simulink model "verification_simulink"  (R2015a)
settings: Solver=ode3  StartTime=0.0  StopTime=T_sim_length  FixedStep=T_sim  RelTol=1e-3
values from neighbouring files (symbols this model uses):
  Ad = sys_discrete.a + L * C + sys_discrete.b * K    [example_integrator.m]    (also in param_pendulum_calc.m)
  Ap = [0, 1; 0, 0]    [example_integrator.m]    (also in param_pendulum.m = [0, 1; upright * omega0 ^ 2, -2 * xi * omega0])
  Bd = -L    [example_integrator.m]    (also in param_pendulum_calc.m)
  Bp = [0; 1]    [example_integrator.m]    (also in example_mimo.m = [Bp, Bp]; param_pendulum.m = [0; omega0 / 9.81])
  C = [1, 0]    [example_integrator.m]    (also in example_mimo.m = [C; C]; param_pendulum.m)
  Cd = K    [example_integrator.m]    (also in param_pendulum_calc.m)
  delay_u_sim_is_random = 0    [example_integrator.m]    (also in example_pendulum_static_delay.m = false; example_pendulum_varying_delay.m = false; param_pendulum_timevarying.m = false)
  delay_y_sim_is_random = 0    [example_integrator.m]    (also in example_pendulum_static_delay.m = false; example_pendulum_varying_delay.m = true; param_pendulum_timevarying.m = false)
  Gp = [0; 1]    [example_integrator.m]    (also in param_pendulum.m)
  N_p = 1e-2    (= 0.01)    [example_integrator.m]    (also in example_mimo.m = blkdiag(N_p, N_p) * 2; param_pendulum.m = 1e-06)
  Q_tilde = [0.00968, 0; 0, 0.0470]    [example_integrator.m]    (also in param_pendulum.m = 550 * eye(2))
  R_tilde = 0.768    [example_integrator.m]    (also in example_mimo.m = blkdiag(R_tilde, R_tilde) * 2; param_pendulum.m = 0.8)
  T = 1    [example_integrator.m]    (also in param_pendulum.m = 0.2)
  T_sim = T * 1e-3    (= 0.001)    [example_integrator.m]    (also in param_pendulum.m = 0.0001)
libraries: simulink x9, dspsigops x2
settings Model: ExtModeTrigDuration=100  Creator=ak22emur  LastModifiedBy=ak22emur
settings DataIOCC: LimitDataPoints=off  SaveFormat=StructureWithTime  SaveOutput=off  SignalLogging=off  DSMLogging=off  VisualizeSimOutput=off  SaveTime=off  StateSaveName=tmp_raccel_xout  SignalLoggingName=tmp_raccel_logsout
settings OptimizationCC: InlineParams=on  InlineInvariantSignals=on  EfficientMapNaN2IntZero=off  SimCompilerOptimization=on
settings HardwareCC: TargetLongLongMode=on  TargetIntDivRoundTo=Zero  TargetEndianess=LittleEndian  TargetHWDeviceType=MATLAB Host  ProdEqTarget=off
settings RTWCC: SystemTargetFile=raccel.tlc  TemplateMakefile=raccel_default_tmf  RTWVerbose=off  RTWUseSimCustomCode=on
settings CodeAppCC: GenerateComments=off  MaxIdLength=128  SimulinkBlockComments=off
settings RaccelTargetCC: ERTMultiwordTypeDef=System defined  ERTMultiwordLength=256  GeneratePreprocessorConditionals=Disable all  ERTFirstTimeCompliant=off  MultiInstanceERTCode=off  ENABLE_SLEXEC_SSBRIDGE=0  RTWCAPIParams=off

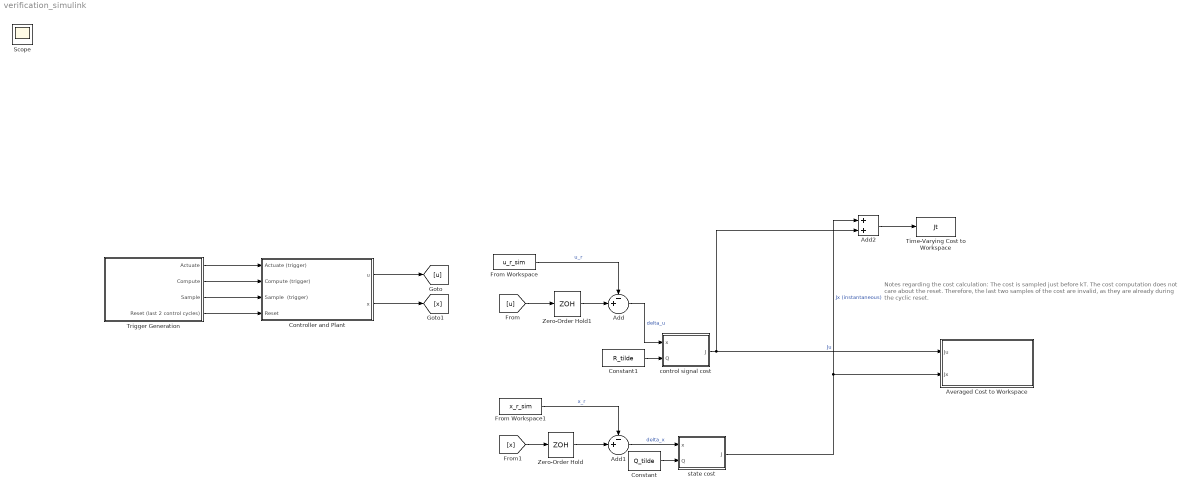
== system verification_simulink ==
  note: Notes regarding the cost calculation:
      | The cost is sampled just before kT.
      | The cost computation does not care about the reset. Therefore, the last two samples of the cost are invalid, as they are already during the cyclic reset.
  Add : Sum  Inputs=-+|
  Add1 : Sum  Inputs=-+|
  Add2 : Sum
  Averaged Cost to Workspace : Subsystem
  Constant : Constant  Value=Q_tilde
  Constant1 : Constant  Value=R_tilde
  Controller and Plant : Subsystem
  From Workspace : FromWorkspace  VariableName=u_r_sim  SampleTime=T  Interpolate=off  OutputAfterFinalValue=Cyclic repetition
  From Workspace1 : FromWorkspace  VariableName=x_r_sim  SampleTime=T  Interpolate=off  OutputAfterFinalValue=Cyclic repetition
  Time-Varying Cost to Workspace : ToWorkspace  VariableName=Jt  SampleTime=T
  Trigger Generation : Subsystem
  Zero-Order Hold : ZeroOrderHold  SampleTime=T
  Zero-Order Hold1 : ZeroOrderHold  SampleTime=T
  control signal cost : MATLAB Function  TreatAsAtomicUnit=on
  state cost : MATLAB Function  TreatAsAtomicUnit=on
  Scope : Scope
      settings: YMin=0  YMax=1.4
  wires:
  Constant/1 -> state cost/2(Q)
  state cost/1(J) -> Averaged Cost to Workspace/2(Jx), Add2/1  "Jx (instantaneous)"
  Constant1/1 -> control signal cost/2(Q)
  control signal cost/1(J) -> Add2/2, Averaged Cost to Workspace/1(Ju)  "Ju"
  [u] -> Zero-Order Hold1/1
  Add2/1 -> Time-Varying Cost to Workspace/1
  Trigger Generation/1(Actuate) -> Controller and Plant/1(Actuate (trigger))
  Trigger Generation/2(Compute) -> Controller and Plant/2(Compute (trigger))
  Trigger Generation/3(Sample) -> Controller and Plant/3(Sample  (trigger))
  Controller and Plant/1(u) -> [u]
  Controller and Plant/2(x) -> [x]
  Trigger Generation/4(Reset (last 2 control cycles)) -> Controller and Plant/4(Reset)
  Add/1 -> control signal cost/1(x)  "delta_u"
  Zero-Order Hold1/1 -> Add/2
  From Workspace/1 -> Add/1  "u_r"
  Add1/1 -> state cost/1(x)  "delta_x"
  [x] -> Zero-Order Hold/1
  From Workspace1/1 -> Add1/1  "x_r"
  Zero-Order Hold/1 -> Add1/2

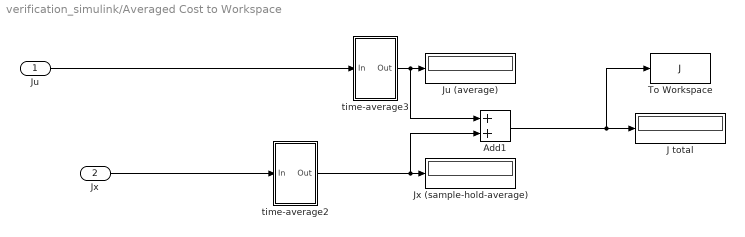
== system verification_simulink/Averaged Cost to Workspace ==
  Ju : Inport
  Jx : Inport  Port=2
  Add1 : Sum
  J total : Display
  Ju (average) : Display
  Jx (sample-hold-average) : Display
  To Workspace : ToWorkspace  VariableName=J  SampleTime=-1
      settings: MaxDataPoints=1
  time-average2 : Subsystem
  time-average3 : Subsystem
  wires:
  time-average3/1(Out) -> Add1/1, Ju (average)/1
  Add1/1 -> To Workspace/1, J total/1
  time-average2/1(Out) -> Add1/2, Jx (sample-hold-average)/1
  Ju/1 -> time-average3/1(In)
  Jx/1 -> time-average2/1(In)

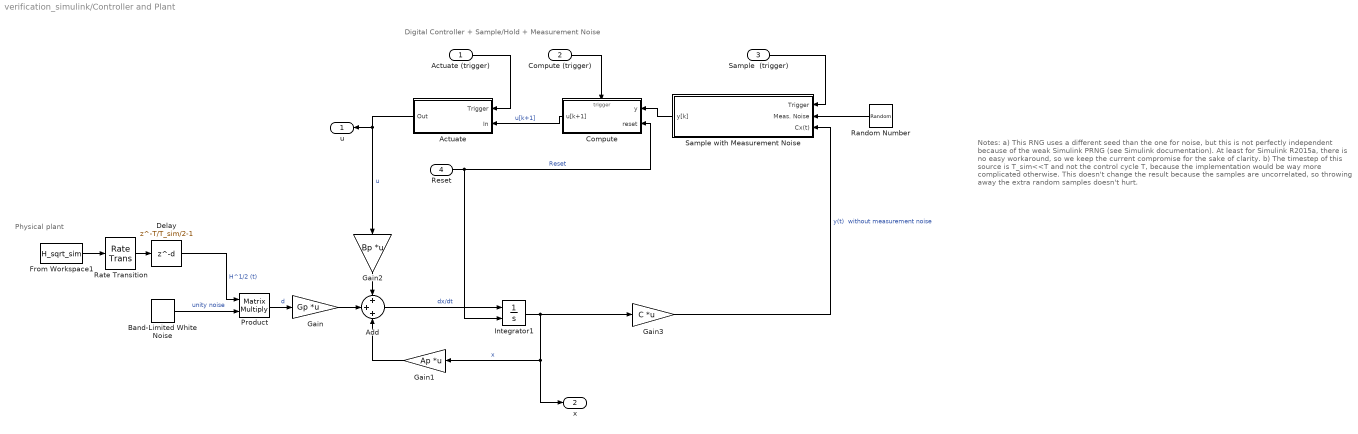
== system verification_simulink/Controller and Plant ==
  note: Digital Controller + Sample/Hold + Measurement Noise
  note: Physical plant
  note: Notes:
      | a) This RNG uses a different seed than the one for noise,
      | but this is not perfectly independent because of the weak Simulink PRNG
      | (see Simulink documentation).
      | At least for Simulink R2015a, there is no easy workaround, so we keep the current compromise for the sake of clarity.
      | b) The timestep of this source is T_sim<<T and not the control cycle T, because the implementation would be way more complicated otherwise.
      | This doesn't change the result because the samples are uncorrelated, so throwing away the extra random samples doesn't hurt.
  Actuate (trigger) : Inport
  Compute (trigger) : Inport  Port=2
  Sample  (trigger) : Inport  Port=3
  Reset : Inport  Port=4
  Actuate : Subsystem  TreatAsAtomicUnit=on
  Add : Sum  Inputs=+++
  Band-Limited White Noise : simulink/Sources/Band-Limited White Noise  Cov=ones(size(Gp,2), 1)  Ts=T_sim  seed=[23341]
  Compute : Subsystem  TreatAsAtomicUnit=on
  Delay : Delay  DelayLength=T/T_sim/2-1
  From Workspace1 : FromWorkspace  VariableName=H_sqrt_sim  SampleTime=T  Interpolate=off  OutputAfterFinalValue=Cyclic repetition
  Gain : Gain  Gain=Gp  Multiplication=Matrix(K*u)
  Gain1 : Gain  Gain=Ap  Multiplication=Matrix(K*u)
  Gain2 : Gain  Gain=Bp  Multiplication=Matrix(K*u)
  Gain3 : Gain  Gain=C  Multiplication=Matrix(K*u)
  Integrator1 : Integrator  ExternalReset=level
  Product : Product  Multiplication=Matrix(*)
  Random Number : RandomNumber  Variance=diag(N_p)  Seed=13379812+[1:length(N_p)]  SampleTime=T_sim
  Rate Transition : RateTransition
  Sample with Measurement Noise : Subsystem  TreatAsAtomicUnit=on
  u : Outport
  x : Outport  Port=2
  wires:
  Gain3/1 -> Sample with Measurement Noise/3(Cx(t))  "y(t)  without measurement noise"
  Gain/1 -> Add/2
  Add/1 -> Integrator1/1  "dx/dt"
  Actuate/1(Out) -> u/1, Gain2/1  "u"
  Gain2/1 -> Add/1
  Compute (trigger)/1 -> Compute/Trigger
  Actuate (trigger)/1 -> Actuate/1(Trigger)
  Integrator1/1 -> x/1, Gain1/1, Gain3/1  "x"
  Compute/1(u[k+1]) -> Actuate/2(In)  "u[k+1]"
  Gain1/1 -> Add/3
  Reset/1 -> Compute/2(reset), Integrator1/2  "Reset"
  Sample  (trigger)/1 -> Sample with Measurement Noise/1(Trigger)
  Random Number/1 -> Sample with Measurement Noise/2(Meas. Noise)
  Sample with Measurement Noise/1(y[k]) -> Compute/1(y)
  Product/1 -> Gain/1  "d"
  Band-Limited White Noise/1 -> Product/2  "unity noise"
  From Workspace1/1 -> Rate Transition/1
  Rate Transition/1 -> Delay/1
  Delay/1 -> Product/1  "H^1/2 (t)"

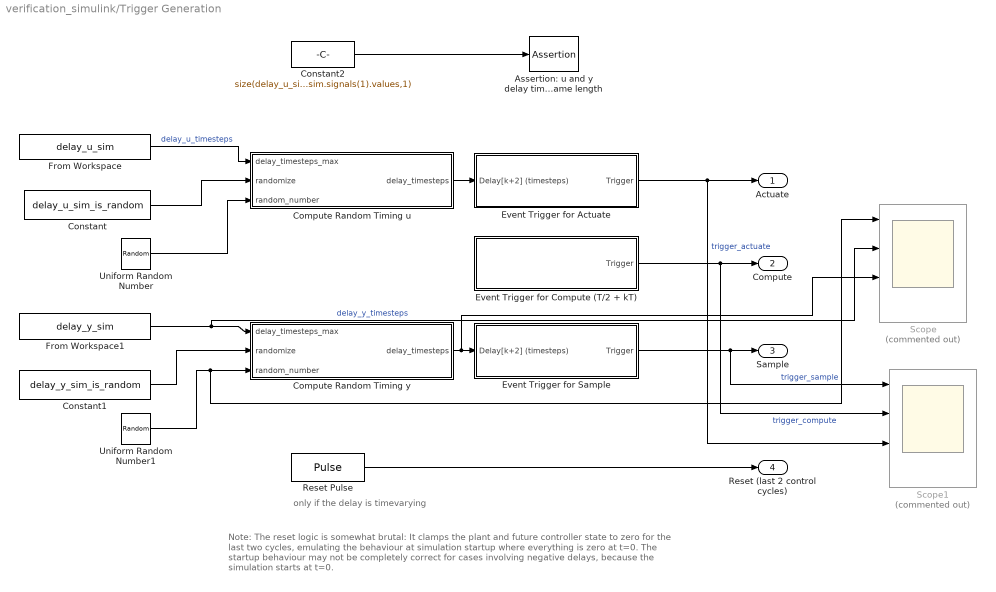
== system verification_simulink/Trigger Generation ==
  note: only if the delay is timevarying
  note: Note: The reset logic is somewhat brutal: It clamps the plant and future controller state to zero for the last two cycles, emulating the behaviour at simulation startup where everything is zero at t=0.
      | The startup behaviour may not be completely correct for cases involving negative delays, because the simulation starts at t=0.
  Assertion: u and y delay timeseries have same length : Assertion
  Compute Random Timing u : MATLAB Function  TreatAsAtomicUnit=on
  Compute Random Timing y : MATLAB Function  TreatAsAtomicUnit=on
  Constant : Constant  Value=delay_u_sim_is_random
  Constant1 : Constant  Value=delay_y_sim_is_random
  Constant2 : Constant  Value=size(delay_u_sim.signals(1).values,1)==size(delay_y_sim.signals(1).values,1)
  Event Trigger for Actuate : Subsystem
  Event Trigger for Compute (T/2 + kT) : Subsystem
  Event Trigger for Sample : Subsystem
  From Workspace : FromWorkspace  VariableName=delay_u_sim  SampleTime=T  Interpolate=off  OutputAfterFinalValue=Cyclic repetition
  From Workspace1 : FromWorkspace  VariableName=delay_y_sim  SampleTime=T  Interpolate=off  OutputAfterFinalValue=Cyclic repetition
  Reset Pulse : DiscretePulseGenerator  Period=size(delay_u_sim.signals(1).values,1)*T/T_sim + T_sim_length/T_sim*(1==size(delay_u_sim.signals(1).values,1))  PulseWidth=2*T/T_sim  PhaseDelay=-2*T/T_sim  SampleTime=T_sim
  Scope : Scope  Commented=on  NumInputPorts=4
      settings: YMin=-5~-5~-5~-5  YMax=5~5~5~5  SaveName=ScopeData2
  Scope1 : Scope  Commented=on  NumInputPorts=4
      settings: YMin=-5~-5~-5~-5  YMax=5~5~5~5  SaveName=ScopeData3
  Uniform Random Number : UniformRandomNumber  Minimum=0  Seed=1000+[1:size(Bp,2)]  SampleTime=T
  Uniform Random Number1 : UniformRandomNumber  Minimum=0  Seed=2000+[1:size(C,1)]  SampleTime=T
  Actuate : Outport
  Compute : Outport  Port=2
  Sample : Outport  Port=3
  Reset (last 2 control cycles) : Outport  Port=4
  wires:
  Event Trigger for Compute (T/2 + kT)/1(Trigger) -> Scope1/2, Compute/1  "trigger_compute"
  From Workspace1/1 -> Scope/2, Compute Random Timing y/1(delay_timesteps_max)  "delay_y_timesteps"
  From Workspace/1 -> Compute Random Timing u/1(delay_timesteps_max)  "delay_u_timesteps"
  Event Trigger for Actuate/1(Trigger) -> Scope1/3, Actuate/1  "trigger_actuate"
  Constant2/1 -> Assertion: u and y delay timeseries have same length/1
  Event Trigger for Sample/1(Trigger) -> Scope1/1, Sample/1  "trigger_sample"
  Reset Pulse/1 -> Reset (last 2 control cycles)/1
  Compute Random Timing u/1(delay_timesteps) -> Event Trigger for Actuate/1(Delay[k+2] (timesteps))
  Constant/1 -> Compute Random Timing u/2(randomize)
  Uniform Random Number/1 -> Compute Random Timing u/3(random_number)
  Compute Random Timing y/1(delay_timesteps) -> Scope/3, Event Trigger for Sample/1(Delay[k+2] (timesteps))
  Uniform Random Number1/1 -> Scope/1, Compute Random Timing y/3(random_number)
  Constant1/1 -> Compute Random Timing y/2(randomize)

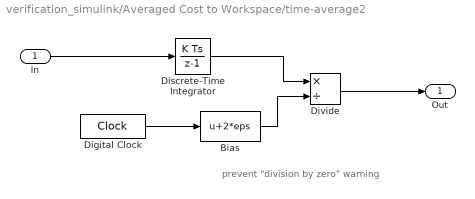
== system verification_simulink/Averaged Cost to Workspace/time-average2 ==
  note: prevent "division by zero" warning
  In : Inport
  Bias : Bias  Bias=2*eps
  Digital Clock : DigitalClock  SampleTime=T
  Discrete-Time Integrator : DiscreteIntegrator  InitialConditionSetting=State (most efficient)  SampleTime=-1
  Divide : Product  Inputs=*/
  Out : Outport
  wires:
  Bias/1 -> Divide/2
  Divide/1 -> Out/1
  Digital Clock/1 -> Bias/1
  Discrete-Time Integrator/1 -> Divide/1
  In/1 -> Discrete-Time Integrator/1

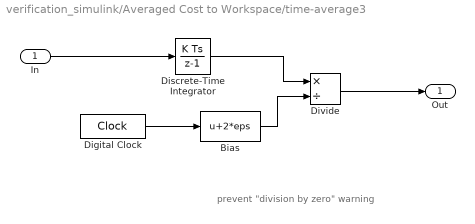
== system verification_simulink/Averaged Cost to Workspace/time-average3 ==
  note: prevent "division by zero" warning
  In : Inport
  Bias : Bias  Bias=2*eps
  Digital Clock : DigitalClock  SampleTime=T
  Discrete-Time Integrator : DiscreteIntegrator  InitialConditionSetting=State (most efficient)  SampleTime=T
  Divide : Product  Inputs=*/
  Out : Outport
  wires:
  Bias/1 -> Divide/2
  Divide/1 -> Out/1
  Digital Clock/1 -> Bias/1
  Discrete-Time Integrator/1 -> Divide/1
  In/1 -> Discrete-Time Integrator/1

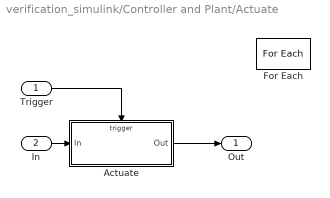
== system verification_simulink/Controller and Plant/Actuate ==
  Trigger : Inport  Partition=on  PartitionDimension=1  PartitionWidth=1
  In : Inport  Port=2  Partition=on  PartitionDimension=1  PartitionWidth=1
  Actuate : Subsystem  TreatAsAtomicUnit=on
  For Each : ForEach  DisableCoverage=on  IndexMode=One-based
  Out : Outport  ConcatenationDimension=1
  wires:
  In/1 -> Actuate/1(In)
  Actuate/1(Out) -> Out/1
  Trigger/1 -> Actuate/Trigger

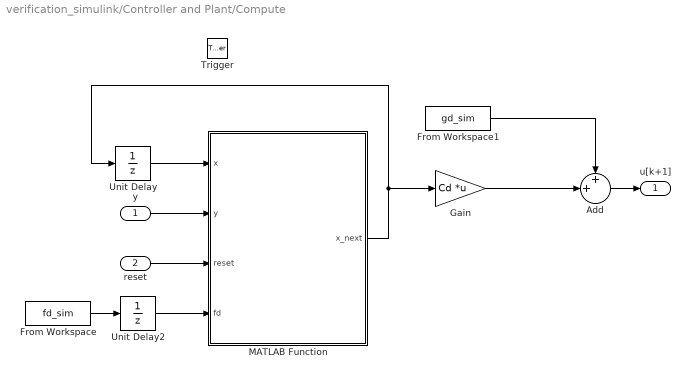
== system verification_simulink/Controller and Plant/Compute ==
  y : Inport
  reset : Inport  Port=2
  Trigger : TriggerPort  PortDimensions=1
  Add : Sum  Inputs=++|
  From Workspace : FromWorkspace  VariableName=fd_sim  Interpolate=off  OutputAfterFinalValue=Cyclic repetition
  From Workspace1 : FromWorkspace  VariableName=gd_sim  Interpolate=off  OutputAfterFinalValue=Cyclic repetition
  Gain : Gain  Gain=Cd  Multiplication=Matrix(K*u)
  MATLAB Function : MATLAB Function  TreatAsAtomicUnit=on
  Unit Delay : UnitDelay  InitialCondition=zeros(1,length(Ad))  SampleTime=-1
  Unit Delay2 : UnitDelay  InitialCondition=zeros(1,length(Ad))  SampleTime=-1
  u[k+1] : Outport
  wires:
  MATLAB Function/1(x_next) -> Unit Delay/1, Gain/1
  y/1 -> MATLAB Function/2(y)
  Unit Delay/1 -> MATLAB Function/1(x)
  reset/1 -> MATLAB Function/3(reset)
  From Workspace/1 -> Unit Delay2/1
  Add/1 -> u[k+1]/1
  Gain/1 -> Add/2
  From Workspace1/1 -> Add/1
  Unit Delay2/1 -> MATLAB Function/4(fd)

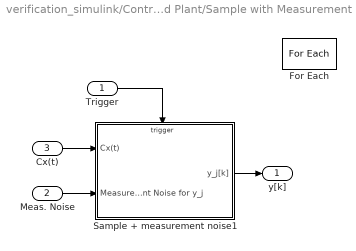
== system verification_simulink/Controller and Plant/Sample with Measurement Noise ==
  Trigger : Inport  Partition=on  PartitionDimension=1  PartitionWidth=1
  Meas. Noise : Inport  Port=2  Partition=on  PartitionDimension=1  PartitionWidth=1
  Cx(t) : Inport  Port=3  Partition=on  PartitionDimension=1  PartitionWidth=1
  For Each : ForEach  DisableCoverage=on  IndexMode=One-based
  Sample + measurement noise1 : Subsystem  TreatAsAtomicUnit=on
  y[k] : Outport  ConcatenationDimension=1
  wires:
  Trigger/1 -> Sample + measurement noise1/Trigger
  Sample + measurement noise1/1(y_j[k]) -> y[k]/1
  Cx(t)/1 -> Sample + measurement noise1/1(Cx(t))
  Meas. Noise/1 -> Sample + measurement noise1/2(Measurement Noise for y_j)

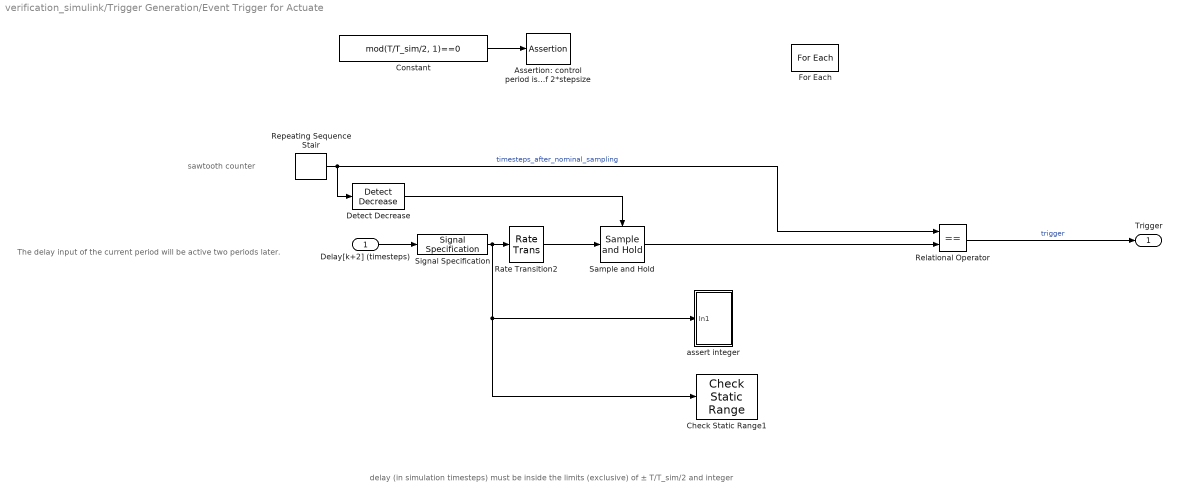
== system verification_simulink/Trigger Generation/Event Trigger for Actuate ==
  note: The delay input of the current period will be active two periods later.
  note: sawtooth counter
  note: delay (in simulation timesteps) must be inside the limits (exclusive) of ± T/T_sim/2
      | and integer
  Delay[k+2] (timesteps) : Inport  Partition=on  PartitionDimension=1  PartitionWidth=1
  Assertion: control period is multiple of 2*stepsize : Assertion
  Check Static Range1 : simulink/Model Verification/Check  Static Range  Description=-T/T_sim/2 < u < T/T_sim/2  max=T/T_sim/2  max_included=off  min=-T/T_sim/2  min_included=off  enabled=on  stopWhenAssertionFail=on  export=off  icon=graphic
  Constant : Constant  Value=mod(T/T_sim/2, 1)==0
  Detect Decrease : simulink/Logic and Bit Operations/Detect Decrease  vinit=inf  InputProcessing=Inherited  OutDataTypeStr=boolean
  For Each : ForEach  DisableCoverage=on  IndexMode=One-based
  Rate Transition2 : RateTransition  OutPortSampleTime=T_sim
  Relational Operator : RelationalOperator  Operator===  OutDataTypeStr=boolean
  Repeating Sequence Stair : simulink/Sources/Repeating Sequence Stair  OutValues=circshift((0:(T/T_sim - 1)) - (T/T_sim/2), [0, T/T_sim/2])  tsamp=T_sim  OutMin=[]  OutMax=[]  OutDataTypeStr=double  OutputDataTypeScalingMode=double  OutDataType=fixdt(0,8)  ConRadixGroup=Best Precision: Vector-wise  OutScaling=2^-12
  Sample and Hold : dspsigops/Sample and Hold  trig=Rising edge  initCond=0  latchinput=off
  Signal Specification : SignalSpecification  Dimensions=1
  assert integer : Subsystem
  Trigger : Outport  ConcatenationDimension=1
  wires:
  Signal Specification/1 -> Rate Transition2/1, assert integer/1(In1), Check Static Range1/1
  Rate Transition2/1 -> Sample and Hold/1
  Detect Decrease/1 -> Sample and Hold/Trigger
  Delay[k+2] (timesteps)/1 -> Signal Specification/1
  Sample and Hold/1 -> Relational Operator/2
  Repeating Sequence Stair/1 -> Relational Operator/1, Detect Decrease/1  "timesteps_after_nominal_sampling"
  Relational Operator/1 -> Trigger/1  "trigger"
  Constant/1 -> Assertion: control period is multiple of 2*stepsize/1

== system verification_simulink/Trigger Generation/Event Trigger for Compute (T//2 + kT) ==
  note: sawtooth counter
  Detect Decrease : simulink/Logic and Bit Operations/Detect Decrease  vinit=inf  InputProcessing=Inherited  OutDataTypeStr=boolean
  Repeating Sequence Stair : simulink/Sources/Repeating Sequence Stair  OutValues=circshift((0:(T/T_sim - 1)) - (T/T_sim/2), [0, T/T_sim/2])  tsamp=T_sim  OutMin=[]  OutMax=[]  OutDataTypeStr=double  OutputDataTypeScalingMode=double  OutDataType=fixdt(0,8)  ConRadixGroup=Best Precision: Vector-wise  OutScaling=2^-12
  Trigger : Outport
  wires:
  Repeating Sequence Stair/1 -> Detect Decrease/1  "timesteps_after_nominal_sampling"
  Detect Decrease/1 -> Trigger/1

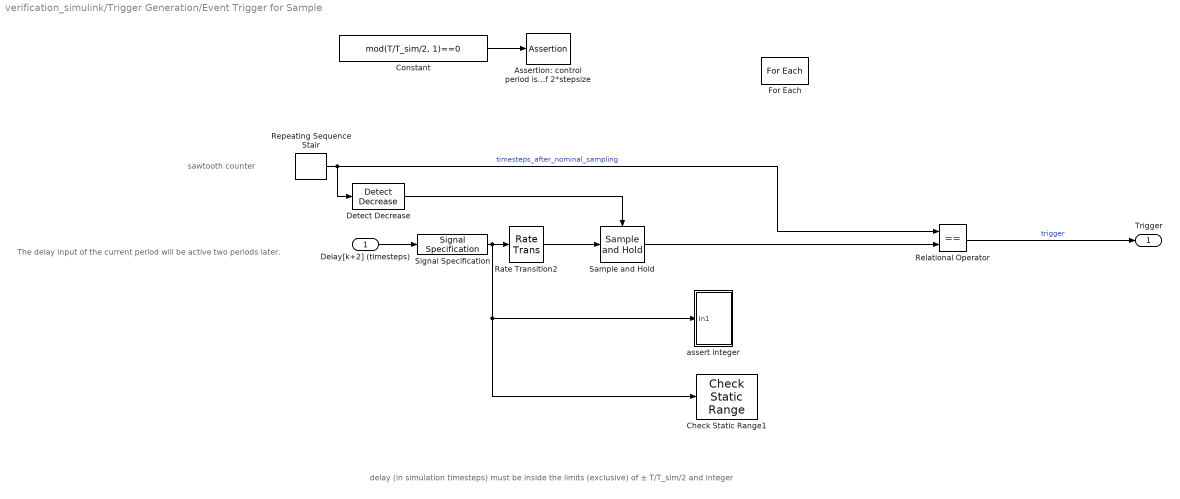
== system verification_simulink/Trigger Generation/Event Trigger for Sample ==
  note: delay (in simulation timesteps) must be inside the limits (exclusive) of ± T/T_sim/2
      | and integer
  note: sawtooth counter
  note: The delay input of the current period will be active two periods later.
  Delay[k+2] (timesteps) : Inport  Partition=on  PartitionDimension=1  PartitionWidth=1
  Assertion: control period is multiple of 2*stepsize : Assertion
  Check Static Range1 : simulink/Model Verification/Check  Static Range  Description=-T/T_sim/2 < u < T/T_sim/2  max=T/T_sim/2  max_included=off  min=-T/T_sim/2  min_included=off  enabled=on  stopWhenAssertionFail=on  export=off  icon=graphic
  Constant : Constant  Value=mod(T/T_sim/2, 1)==0
  Detect Decrease : simulink/Logic and Bit Operations/Detect Decrease  vinit=inf  InputProcessing=Inherited  OutDataTypeStr=boolean
  For Each : ForEach  DisableCoverage=on  IndexMode=One-based
  Rate Transition2 : RateTransition  OutPortSampleTime=T_sim
  Relational Operator : RelationalOperator  Operator===  OutDataTypeStr=boolean
  Repeating Sequence Stair : simulink/Sources/Repeating Sequence Stair  OutValues=circshift((0:(T/T_sim - 1)) - (T/T_sim/2), [0, T/T_sim/2])  tsamp=T_sim  OutMin=[]  OutMax=[]  OutDataTypeStr=double  OutputDataTypeScalingMode=double  OutDataType=fixdt(0,8)  ConRadixGroup=Best Precision: Vector-wise  OutScaling=2^-12
  Sample and Hold : dspsigops/Sample and Hold  trig=Rising edge  initCond=0  latchinput=off
  Signal Specification : SignalSpecification  Dimensions=1
  assert integer : Subsystem
  Trigger : Outport  ConcatenationDimension=1
  wires:
  Constant/1 -> Assertion: control period is multiple of 2*stepsize/1
  Relational Operator/1 -> Trigger/1  "trigger"
  Repeating Sequence Stair/1 -> Detect Decrease/1, Relational Operator/1  "timesteps_after_nominal_sampling"
  Sample and Hold/1 -> Relational Operator/2
  Delay[k+2] (timesteps)/1 -> Signal Specification/1
  Detect Decrease/1 -> Sample and Hold/Trigger
  Rate Transition2/1 -> Sample and Hold/1
  Signal Specification/1 -> Check Static Range1/1, assert integer/1(In1), Rate Transition2/1

== system verification_simulink/Controller and Plant/Actuate/Actuate ==
  In : Inport
  Trigger : TriggerPort  PortDimensions=1
  Out : Outport
  wires:
  In/1 -> Out/1

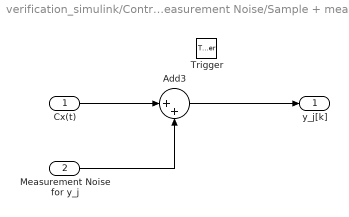
== system verification_simulink/Controller and Plant/Sample with Measurement Noise/Sample + measurement noise1 ==
  Cx(t) : Inport
  Measurement Noise for y_j : Inport  Port=2
  Trigger : TriggerPort  PortDimensions=1
  Add3 : Sum  Inputs=|++
  y_j[k] : Outport
  wires:
  Measurement Noise for y_j/1 -> Add3/2
  Add3/1 -> y_j[k]/1
  Cx(t)/1 -> Add3/1

== system verification_simulink/Trigger Generation/Event Trigger for Actuate/assert integer ==
  In1 : Inport
  Assertion : Assertion
  MATLAB Function : MATLAB Function  TreatAsAtomicUnit=on
  wires:
  MATLAB Function/1(y) -> Assertion/1
  In1/1 -> MATLAB Function/1(u)

== system verification_simulink/Trigger Generation/Event Trigger for Sample/assert integer ==
  In1 : Inport
  Assertion : Assertion
  MATLAB Function : MATLAB Function  TreatAsAtomicUnit=on
  wires:
  In1/1 -> MATLAB Function/1(u)
  MATLAB Function/1(y) -> Assertion/1

== matlab function verification_simulink/control signal cost ==
  data: x input; J output; Q input
function J = cost(x,Q)
%#codegen

J=x'*Q*x;

== matlab function verification_simulink/state cost ==
  data: x input; J output; Q input
function J = cost(x,Q)
%#codegen

J=x'*Q*x;

== matlab function verification_simulink/Trigger Generation/Event Trigger for Actuate/assert integer/MATLAB Function ==
  data: u input; y output
function y = isInteger(u)
%#codegen

y = mod(u,1)==0;

== matlab function verification_simulink/Trigger Generation/Event Trigger for Sample/assert integer/MATLAB Function ==
  data: u input; y output
function y = isInteger(u)
%#codegen

y = mod(u,1)==0;

== matlab function verification_simulink/Controller and Plant/Compute/MATLAB Function ==
  data: x input; y input; reset input; x_next output; Ad parameter; Bd parameter; fd input
function x_next = fcn(x, y, reset, Ad, Bd, fd)
%#codegen
x_next = Ad * x + Bd * y + fd;
if reset
    x_next = 0*x_next;
end

== matlab function verification_simulink/Trigger Generation/Compute Random Timing u ==
  data: delay_timesteps_max input; delay_timesteps output; randomize input; random_number input
function delay_timesteps = fcn(delay_timesteps_max, randomize, random_number)
%#codegen

% 0 < random_number(i) < 1.
if randomize
    delay_timesteps = round(delay_timesteps_max .* random_number);
else
    delay_timesteps = delay_timesteps_max;
end

== matlab function verification_simulink/Trigger Generation/Compute Random Timing y ==
  data: delay_timesteps_max input; delay_timesteps output; randomize input; random_number input
function delay_timesteps = fcn(delay_timesteps_max, randomize, random_number)
%#codegen

% 0 < random_number(i) < 1.
if randomize
    delay_timesteps = round(delay_timesteps_max .* random_number);
else
    delay_timesteps = delay_timesteps_max;
end
